simulink model "simulink model of all the components of the car"  (R2024a)
settings: Solver=VariableStepAuto  StartTime=0.0  StopTime=10.0  RelTol=1e-3
undefined symbols (not defined in the file or in its folder): canChannel
libraries: canlib x3, canmsglib x2

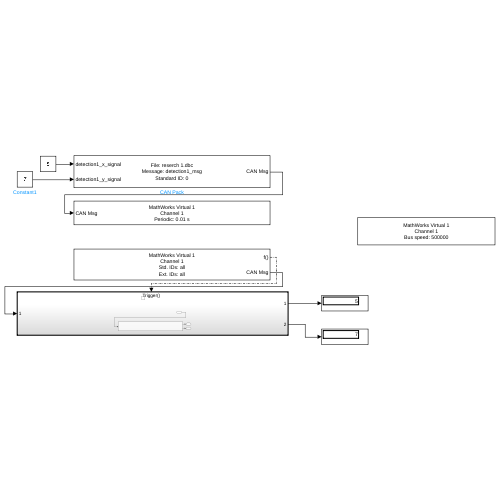
[thumbnail: Simulink's stored preview of the top-level diagram]
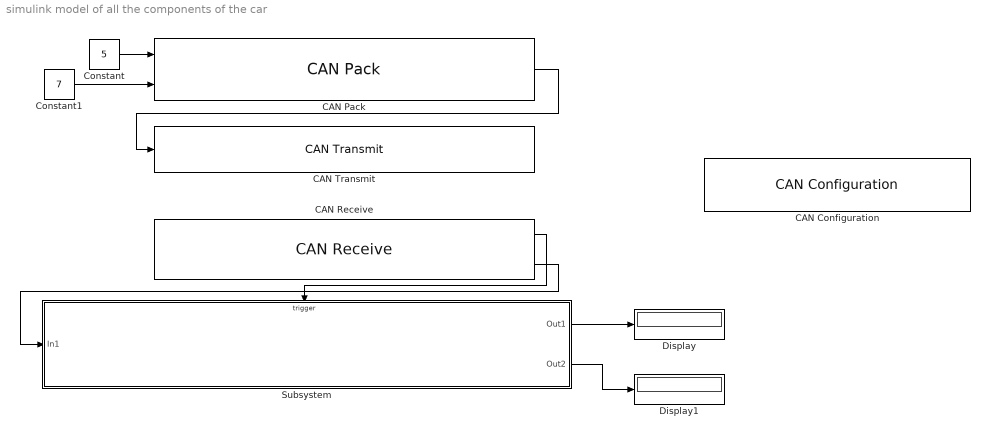
== system simulink model of all the components of the car ==
  CAN Configuration : canlib/CAN Configuration  BlockHandle=154.0002  Device=MathWorks Virtual 1 (Channel 1)  DeviceMenu=MathWorks Virtual 1 (Channel 1)  ObjConstructor=canChannel('MathWorks', 'Virtual 1', 1)  BusSpeed=500000  EnableBitParameters=off  AckMode=Normal
  CAN Pack : canmsglib/CAN Pack  CANdbFile=/MATLAB Drive/research/reserch 1.dbc  MsgList=detection1_msg  MsgName=detection1_msg  MsgIDType=Standard (11-bit identifier)  MsgIdentifier=0  MsgLength=2  Remote=off  ApplyMinMax=off  BusOutput=off  SignalInfo={'detection1_x_signal','0','8','LE','signed','Standard','0','1','0','-Inf','Inf';'detection1_y_signal','8','8','LE','signed','Standard','0','1','0','-Inf','Inf'}
      settings: LibrarySourceBlock=canlib/CAN Pack  DataFormat=CANdb specified signals
  CAN Receive : canlib/CAN Receive  BlockHandle=158.0002  Device=MathWorks Virtual 1 (Channel 1)  DeviceMenu=MathWorks Virtual 1 (Channel 1)  ObjConstructor=canChannel('MathWorks', 'Virtual 1', 1)  EnableStandardIDsFilter=off  StdIDsCombo=Allow all  StandardIDs=0  EnableExtendedIDsFilter=off  ExtIDsCombo=Allow all  ExtendedIDs=0  SampleTime=0.01  MsgsPerTimestep=all  InternalFilterUpdateStatus=on  BusOutput=off
  CAN Transmit : canlib/CAN Transmit  BlockHandle=161.0002  Device=MathWorks Virtual 1 (Channel 1)  DeviceMenu=MathWorks Virtual 1 (Channel 1)  ObjConstructor=canChannel('MathWorks', 'Virtual 1', 1)  EnableEventTransmit=off  EnablePeriodicTransmit=on  MessagePeriod=0.01
  Constant : Constant  Value=5
  Constant1 : Constant  Value=7
  Display : Display
  Display1 : Display
  Subsystem : Subsystem
  wires:
  Constant/1 -> CAN Pack/1
  Constant1/1 -> CAN Pack/2
  CAN Pack/1 -> CAN Transmit/1
  CAN Receive/2 -> Subsystem/1(In1)
  CAN Receive/1 -> Subsystem/Trigger
  Subsystem/1(Out1) -> Display/1
  Subsystem/2(Out2) -> Display1/1

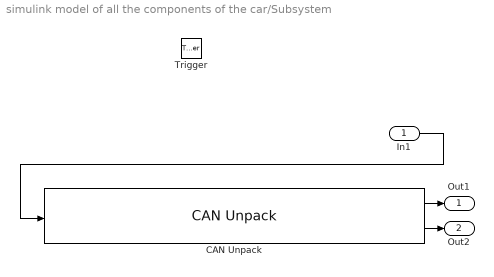
== system simulink model of all the components of the car/Subsystem ==
  In1 : Inport
  Trigger : TriggerPort  TriggerType=function-call  VariantControl=(inherit)  PortDimensions=1
  CAN Unpack : canmsglib/CAN Unpack  CANdbFile=/MATLAB Drive/research/reserch 1.dbc  MsgList=detection1_msg  MsgName=detection1_msg  MsgIDType=Standard (11-bit identifier)  MsgIdentifier=0  MsgLength=2  SignalInfo={'detection1_x_signal','0','8','LE','signed','Standard','0','1','0','-Inf','Inf';'detection1_y_signal','8','8','LE','signed','Standard','0','1','0','-Inf','Inf'}  IDPort=off  TimestampPort=off  ErrorPort=off  RemotePort=off  LengthPort=off  StatusPort=off  ApplyMinMax=off
      settings: LibrarySourceBlock=canlib/CAN Unpack  DataFormat=CANdb specified signals
  Out1 : Outport
  Out2 : Outport  Port=2
  wires:
  In1/1 -> CAN Unpack/1
  CAN Unpack/1 -> Out1/1
  CAN Unpack/2 -> Out2/1
